simulink model "assemblage_19"  (R2016a)
settings: Solver=ode15s  StartTime=0.0  StopTime=1e6  RelTol=1e-3
undefined symbols (not defined in the file or in its folder): W
libraries: simCryogenics_lib x424, nesl_utility x343, fl_lib x9
(part 2 of 3)

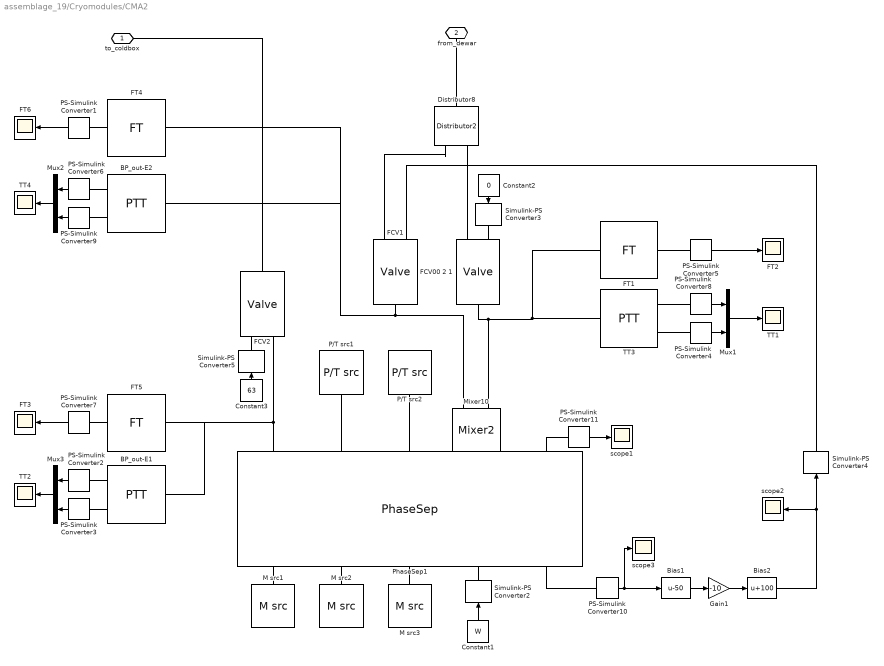
== system assemblage_19/Cryomodules/CMA2 ==
  BP_out-E1 : simCryogenics_lib/Sensors/PTT
  BP_out-E2 : simCryogenics_lib/Sensors/PTT
  Bias1 : Bias  Bias=-50
  Bias2 : Bias  Bias=100
  Constant1 : Constant  Value=W
  Constant2 : Constant  Value=0
  Constant3 : Constant  Value=63
  Distributor8 : simCryogenics_lib/Elements/Distributor2
  FCV00 2 1 : simCryogenics_lib/Elements/Valve  CVmax=0.2  ControlInputMin=0  ControlInputMax=100  Xt=0.86  Rv=100  lin_v=0  lim_v=0  K=2.4e-5 m^1.50000*kg^0.50000/s/bar^0.50000  Cmd_specify=off  Cmd_priority=High  Cmd=0  gamma_specify=off  gamma_priority=High  gamma=0  rho_specify=off  rho_priority=High  rho=0 kg/m^3  Xc_specify=off  Xc_priority=High  Xc=0  X_specify=off  X_priority=High  X=0  Y_specify=off  Y_priority=High  Y=0  CV_specify=off  CV_priority=High  CV=0
  FCV1 : simCryogenics_lib/Elements/Valve  CVmax=1.25  ControlInputMin=0  ControlInputMax=100  Xt=0.86  Rv=150  lin_v=0  lim_v=0  K=2.4e-5 m^1.50000*kg^0.50000/s/bar^0.50000  Cmd_specify=off  Cmd_priority=High  Cmd=0  gamma_specify=off  gamma_priority=High  gamma=0  rho_specify=off  rho_priority=High  rho=0 kg/m^3  Xc_specify=off  Xc_priority=High  Xc=0  X_specify=off  X_priority=High  X=0  Y_specify=off  Y_priority=High  Y=0  CV_specify=off  CV_priority=High  CV=0
  FCV2 : simCryogenics_lib/Elements/Valve  CVmax=1.5  ControlInputMin=0  ControlInputMax=100  Xt=0.86  Rv=100  lin_v=0  lim_v=0  K=2.4e-5 m^1.50000*kg^0.50000/s/bar^0.50000  Cmd_specify=off  Cmd_priority=High  Cmd=0  gamma_specify=off  gamma_priority=High  gamma=0  rho_specify=off  rho_priority=High  rho=0 kg/m^3  Xc_specify=off  Xc_priority=High  Xc=0  X_specify=off  X_priority=High  X=0  Y_specify=off  Y_priority=High  Y=0  CV_specify=off  CV_priority=High  CV=0
  FT1 : simCryogenics_lib/Sensors/FT
  FT2 : Scope
  FT3 : Scope
  FT4 : simCryogenics_lib/Sensors/FT
  FT5 : simCryogenics_lib/Sensors/FT
  FT6 : Scope
  Gain1 : Gain  Gain=-10
  M src1 : simCryogenics_lib/Sources_Sinks/M src  M=0 kg/s
  M src2 : simCryogenics_lib/Sources_Sinks/M src  M=0 kg/s
  M src3 : simCryogenics_lib/Sources_Sinks/M src  M=0 kg/s
  Mixer10 : simCryogenics_lib/Elements/Mixer2
  Mux1 : Mux  Inputs=2
  Mux2 : Mux  Inputs=2
  Mux3 : Mux  Inputs=2
  P/T src1 : simCryogenics_lib/Sources_Sinks/P//T src  P=1.2 bar  T=4.4 K
  P/T src2 : simCryogenics_lib/Sources_Sinks/P//T src  P=1.2 bar  T=4.4 K
  PS-Simulink Converter{1..11} (11 alike) : nesl_utility/PS-Simulink Converter  PhysicalDomain=network_engine_domain  SubClassName=ps_output  LeftPortType=input  RightPortType=output  PseudoPeriodic=off  Frequencies=[]  Unit=1  AffineConversion=off
  PhaseSep1 : simCryogenics_lib/Elements/PhaseSep  Ideal1=1  DeltaT1=0.05 K  N1=10  h1=400 W/K  Ideal2=1  DeltaT2=0.05 K  N2=10  h2=400 W/K  hmax=0.870 m  S=0.0402 m^2  P0=1.25 bar  h0=50  T0=4.5 K
  Simulink-PS Converter{2..5} (4 alike) : nesl_utility/Simulink-PS Converter  PhysicalDomain=network_engine_domain  SubClassName=ps_input  LeftPortType=input  RightPortType=output  PseudoPeriodic=off  Frequencies=[]  NoiseDistribution=none  NoiseParameters=[]  Unit=1  AffineConversion=off  InputFiltering=off  SimscapeFilterOrder=1  InputFilterTimeConstant=0.001  UdotUserProvided=1
  TT1 : Scope
  TT2 : Scope
  TT3 : simCryogenics_lib/Sensors/PTT
  TT4 : Scope
  scope1 : Scope
  scope2 : Scope
  scope3 : Scope
  to_coldbox : PMIOPort  Port=1  Side=Left
  from_dewar : PMIOPort  Port=2  Side=Right
  wires:
  PS-Simulink Converter5/1 -> FT2/1
  PS-Simulink Converter6/1 -> Mux2/1
  Mux3/1 -> TT2/1
  PS-Simulink Converter10/1 -> scope3/1, Bias1/1
  Constant3/1 -> Simulink-PS Converter5/1
  PS-Simulink Converter3/1 -> Mux3/2
  Constant2/1 -> Simulink-PS Converter3/1
  PS-Simulink Converter9/1 -> Mux2/2
  PS-Simulink Converter7/1 -> FT3/1
  PS-Simulink Converter1/1 -> FT6/1
  Gain1/1 -> Bias2/1
  PS-Simulink Converter11/1 -> scope1/1
  Mux2/1 -> TT4/1
  PS-Simulink Converter2/1 -> Mux3/1
  Mux1/1 -> TT1/1
  PS-Simulink Converter4/1 -> Mux1/2
  Bias2/1 -> scope2/1, Simulink-PS Converter4/1
  Constant1/1 -> Simulink-PS Converter2/1
  PS-Simulink Converter8/1 -> Mux1/1
  Bias1/1 -> Gain1/1
  connections:
  Simulink-PS Converter3/RConn1 -- FCV00 2 1/LConn1
  BP_out-E2/RConn2 -- PS-Simulink Converter6/LConn1
  PhaseSep1/RConn2 -- M src2/RConn1
  FCV1/RConn1 -- Mixer10/LConn2 -- FT4/LConn1 -- BP_out-E2/LConn1
  FT1/LConn1 -- TT3/LConn1 -- FCV00 2 1/RConn1 -- Mixer10/LConn1
  P/T src2/RConn1 -- PhaseSep1/LConn3
  TT3/RConn2 -- PS-Simulink Converter4/LConn1
  PS-Simulink Converter1/LConn1 -- FT4/RConn1
  FCV2/LConn1 -- Simulink-PS Converter5/RConn1
  Simulink-PS Converter2/RConn1 -- PhaseSep1/RConn4
  M src3/RConn1 -- PhaseSep1/RConn3
  FCV2/RConn1 -- to_coldbox/RConn1
  PhaseSep1/LConn2 -- P/T src1/RConn1
  FCV00 2 1/LConn2 -- Distributor8/RConn1
  BP_out-E1/RConn2 -- PS-Simulink Converter2/LConn1
  PhaseSep1/LConn4 -- Mixer10/RConn1
  PS-Simulink Converter10/LConn1 -- PhaseSep1/RConn5
  TT3/RConn1 -- PS-Simulink Converter8/LConn1
  FCV2/LConn2 -- PhaseSep1/LConn1 -- BP_out-E1/LConn1 -- FT5/LConn1
  from_dewar/RConn1 -- Distributor8/LConn1
  PS-Simulink Converter11/LConn1 -- PhaseSep1/LConn5
  M src1/RConn1 -- PhaseSep1/RConn1
  BP_out-E2/RConn1 -- PS-Simulink Converter9/LConn1
  PS-Simulink Converter5/LConn1 -- FT1/RConn1
  BP_out-E1/RConn1 -- PS-Simulink Converter3/LConn1
  Simulink-PS Converter4/RConn1 -- FCV1/LConn1
  PS-Simulink Converter7/LConn1 -- FT5/RConn1
  Distributor8/RConn2 -- FCV1/LConn2

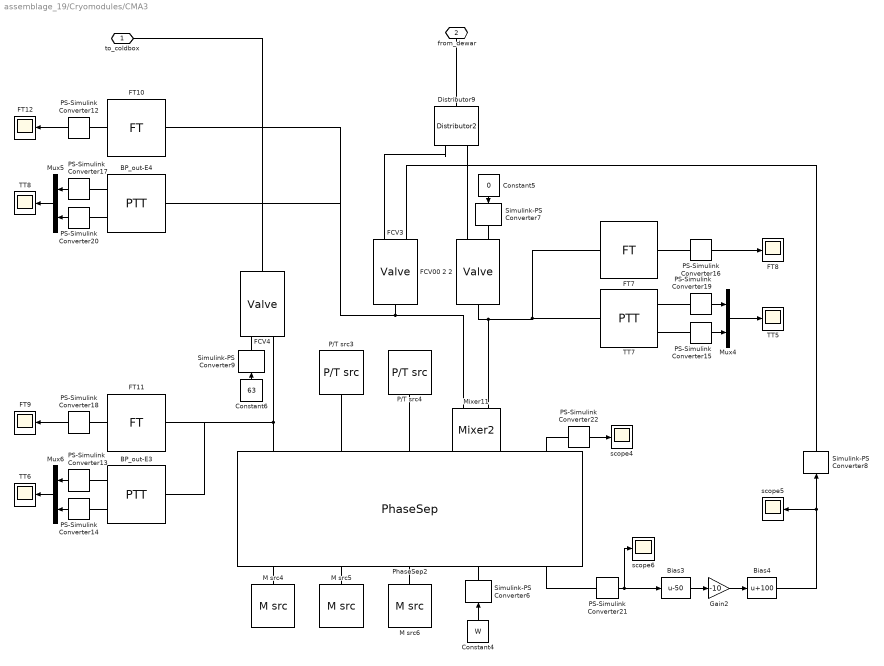
== system assemblage_19/Cryomodules/CMA3 ==
  BP_out-E3 : simCryogenics_lib/Sensors/PTT
  BP_out-E4 : simCryogenics_lib/Sensors/PTT
  Bias3 : Bias  Bias=-50
  Bias4 : Bias  Bias=100
  Constant4 : Constant  Value=W
  Constant5 : Constant  Value=0
  Constant6 : Constant  Value=63
  Distributor9 : simCryogenics_lib/Elements/Distributor2
  FCV00 2 2 : simCryogenics_lib/Elements/Valve  CVmax=0.2  ControlInputMin=0  ControlInputMax=100  Xt=0.86  Rv=100  lin_v=0  lim_v=0  K=2.4e-5 m^1.50000*kg^0.50000/s/bar^0.50000  Cmd_specify=off  Cmd_priority=High  Cmd=0  gamma_specify=off  gamma_priority=High  gamma=0  rho_specify=off  rho_priority=High  rho=0 kg/m^3  Xc_specify=off  Xc_priority=High  Xc=0  X_specify=off  X_priority=High  X=0  Y_specify=off  Y_priority=High  Y=0  CV_specify=off  CV_priority=High  CV=0
  FCV3 : simCryogenics_lib/Elements/Valve  CVmax=1.25  ControlInputMin=0  ControlInputMax=100  Xt=0.86  Rv=150  lin_v=0  lim_v=0  K=2.4e-5 m^1.50000*kg^0.50000/s/bar^0.50000  Cmd_specify=off  Cmd_priority=High  Cmd=0  gamma_specify=off  gamma_priority=High  gamma=0  rho_specify=off  rho_priority=High  rho=0 kg/m^3  Xc_specify=off  Xc_priority=High  Xc=0  X_specify=off  X_priority=High  X=0  Y_specify=off  Y_priority=High  Y=0  CV_specify=off  CV_priority=High  CV=0
  FCV4 : simCryogenics_lib/Elements/Valve  CVmax=1.5  ControlInputMin=0  ControlInputMax=100  Xt=0.86  Rv=100  lin_v=0  lim_v=0  K=2.4e-5 m^1.50000*kg^0.50000/s/bar^0.50000  Cmd_specify=off  Cmd_priority=High  Cmd=0  gamma_specify=off  gamma_priority=High  gamma=0  rho_specify=off  rho_priority=High  rho=0 kg/m^3  Xc_specify=off  Xc_priority=High  Xc=0  X_specify=off  X_priority=High  X=0  Y_specify=off  Y_priority=High  Y=0  CV_specify=off  CV_priority=High  CV=0
  FT10 : simCryogenics_lib/Sensors/FT
  FT11 : simCryogenics_lib/Sensors/FT
  FT12 : Scope
  FT7 : simCryogenics_lib/Sensors/FT
  FT8 : Scope
  FT9 : Scope
  Gain2 : Gain  Gain=-10
  M src4 : simCryogenics_lib/Sources_Sinks/M src  M=0 kg/s
  M src5 : simCryogenics_lib/Sources_Sinks/M src  M=0 kg/s
  M src6 : simCryogenics_lib/Sources_Sinks/M src  M=0 kg/s
  Mixer11 : simCryogenics_lib/Elements/Mixer2
  Mux4 : Mux  Inputs=2
  Mux5 : Mux  Inputs=2
  Mux6 : Mux  Inputs=2
  P/T src3 : simCryogenics_lib/Sources_Sinks/P//T src  P=1.2 bar  T=4.4 K
  P/T src4 : simCryogenics_lib/Sources_Sinks/P//T src  P=1.2 bar  T=4.4 K
  PS-Simulink Converter{12..22} (11 alike) : nesl_utility/PS-Simulink Converter  PhysicalDomain=network_engine_domain  SubClassName=ps_output  LeftPortType=input  RightPortType=output  PseudoPeriodic=off  Frequencies=[]  Unit=1  AffineConversion=off
  PhaseSep2 : simCryogenics_lib/Elements/PhaseSep  Ideal1=1  DeltaT1=0.05 K  N1=10  h1=400 W/K  Ideal2=1  DeltaT2=0.05 K  N2=10  h2=400 W/K  hmax=0.870 m  S=0.0402 m^2  P0=1.25 bar  h0=50  T0=4.5 K
  Simulink-PS Converter{6..9} (4 alike) : nesl_utility/Simulink-PS Converter  PhysicalDomain=network_engine_domain  SubClassName=ps_input  LeftPortType=input  RightPortType=output  PseudoPeriodic=off  Frequencies=[]  NoiseDistribution=none  NoiseParameters=[]  Unit=1  AffineConversion=off  InputFiltering=off  SimscapeFilterOrder=1  InputFilterTimeConstant=0.001  UdotUserProvided=1
  TT5 : Scope
  TT6 : Scope
  TT7 : simCryogenics_lib/Sensors/PTT
  TT8 : Scope
  scope4 : Scope
  scope5 : Scope
  scope6 : Scope
  to_coldbox : PMIOPort  Port=1  Side=Left
  from_dewar : PMIOPort  Port=2  Side=Right
  wires:
  PS-Simulink Converter16/1 -> FT8/1
  Mux6/1 -> TT6/1
  PS-Simulink Converter18/1 -> FT9/1
  PS-Simulink Converter20/1 -> Mux5/2
  PS-Simulink Converter17/1 -> Mux5/1
  Bias4/1 -> scope5/1, Simulink-PS Converter8/1
  Gain2/1 -> Bias4/1
  PS-Simulink Converter14/1 -> Mux6/2
  Constant4/1 -> Simulink-PS Converter6/1
  Constant5/1 -> Simulink-PS Converter7/1
  PS-Simulink Converter19/1 -> Mux4/1
  PS-Simulink Converter13/1 -> Mux6/1
  PS-Simulink Converter12/1 -> FT12/1
  Constant6/1 -> Simulink-PS Converter9/1
  PS-Simulink Converter22/1 -> scope4/1
  PS-Simulink Converter21/1 -> scope6/1, Bias3/1
  Mux4/1 -> TT5/1
  PS-Simulink Converter15/1 -> Mux4/2
  Mux5/1 -> TT8/1
  Bias3/1 -> Gain2/1
  connections:
  BP_out-E4/RConn2 -- PS-Simulink Converter17/LConn1
  FCV4/LConn1 -- Simulink-PS Converter9/RConn1
  BP_out-E3/RConn2 -- PS-Simulink Converter13/LConn1
  FT7/LConn1 -- TT7/LConn1 -- FCV00 2 2/RConn1 -- Mixer11/LConn1
  PS-Simulink Converter18/LConn1 -- FT11/RConn1
  from_dewar/RConn1 -- Distributor9/LConn1
  FCV00 2 2/LConn2 -- Distributor9/RConn1
  PhaseSep2/LConn2 -- P/T src3/RConn1
  FCV3/RConn1 -- Mixer11/LConn2 -- FT10/LConn1 -- BP_out-E4/LConn1
  Simulink-PS Converter6/RConn1 -- PhaseSep2/RConn4
  Simulink-PS Converter7/RConn1 -- FCV00 2 2/LConn1
  FCV4/RConn1 -- to_coldbox/RConn1
  PhaseSep2/RConn2 -- M src5/RConn1
  M src4/RConn1 -- PhaseSep2/RConn1
  FCV4/LConn2 -- PhaseSep2/LConn1 -- BP_out-E3/LConn1 -- FT11/LConn1
  Simulink-PS Converter8/RConn1 -- FCV3/LConn1
  PS-Simulink Converter22/LConn1 -- PhaseSep2/LConn5
  Distributor9/RConn2 -- FCV3/LConn2
  P/T src4/RConn1 -- PhaseSep2/LConn3
  TT7/RConn2 -- PS-Simulink Converter15/LConn1
  TT7/RConn1 -- PS-Simulink Converter19/LConn1
  PS-Simulink Converter16/LConn1 -- FT7/RConn1
  BP_out-E3/RConn1 -- PS-Simulink Converter14/LConn1
  M src6/RConn1 -- PhaseSep2/RConn3
  PS-Simulink Converter12/LConn1 -- FT10/RConn1
  PS-Simulink Converter21/LConn1 -- PhaseSep2/RConn5
  PhaseSep2/LConn4 -- Mixer11/RConn1
  BP_out-E4/RConn1 -- PS-Simulink Converter20/LConn1

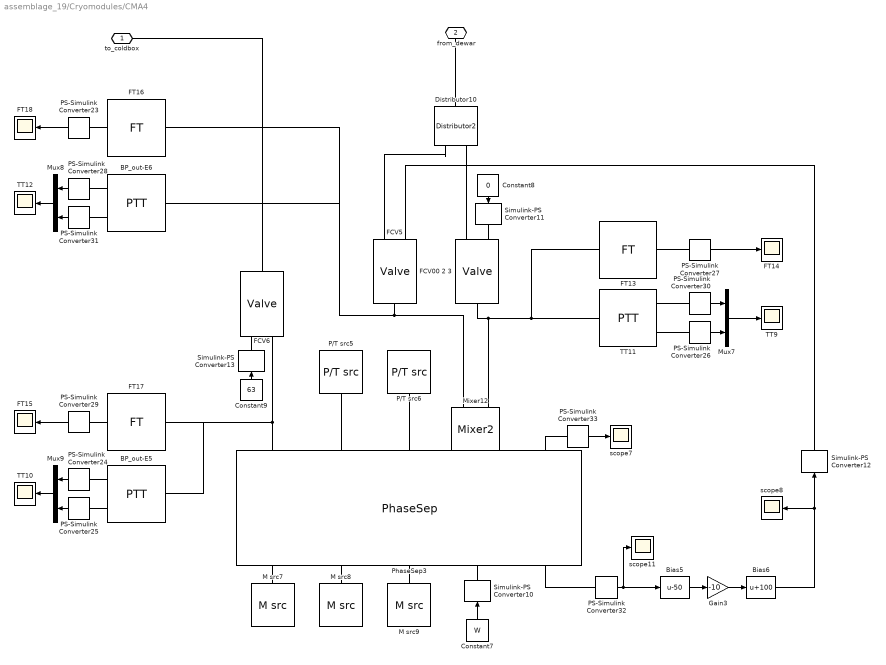
== system assemblage_19/Cryomodules/CMA4 ==
  BP_out-E5 : simCryogenics_lib/Sensors/PTT
  BP_out-E6 : simCryogenics_lib/Sensors/PTT
  Bias5 : Bias  Bias=-50
  Bias6 : Bias  Bias=100
  Constant7 : Constant  Value=W
  Constant8 : Constant  Value=0
  Constant9 : Constant  Value=63
  Distributor10 : simCryogenics_lib/Elements/Distributor2
  FCV00 2 3 : simCryogenics_lib/Elements/Valve  CVmax=0.2  ControlInputMin=0  ControlInputMax=100  Xt=0.86  Rv=100  lin_v=0  lim_v=0  K=2.4e-5 m^1.50000*kg^0.50000/s/bar^0.50000  Cmd_specify=off  Cmd_priority=High  Cmd=0  gamma_specify=off  gamma_priority=High  gamma=0  rho_specify=off  rho_priority=High  rho=0 kg/m^3  Xc_specify=off  Xc_priority=High  Xc=0  X_specify=off  X_priority=High  X=0  Y_specify=off  Y_priority=High  Y=0  CV_specify=off  CV_priority=High  CV=0
  FCV5 : simCryogenics_lib/Elements/Valve  CVmax=1.25  ControlInputMin=0  ControlInputMax=100  Xt=0.86  Rv=150  lin_v=0  lim_v=0  K=2.4e-5 m^1.50000*kg^0.50000/s/bar^0.50000  Cmd_specify=off  Cmd_priority=High  Cmd=0  gamma_specify=off  gamma_priority=High  gamma=0  rho_specify=off  rho_priority=High  rho=0 kg/m^3  Xc_specify=off  Xc_priority=High  Xc=0  X_specify=off  X_priority=High  X=0  Y_specify=off  Y_priority=High  Y=0  CV_specify=off  CV_priority=High  CV=0
  FCV6 : simCryogenics_lib/Elements/Valve  CVmax=1.5  ControlInputMin=0  ControlInputMax=100  Xt=0.86  Rv=100  lin_v=0  lim_v=0  K=2.4e-5 m^1.50000*kg^0.50000/s/bar^0.50000  Cmd_specify=off  Cmd_priority=High  Cmd=0  gamma_specify=off  gamma_priority=High  gamma=0  rho_specify=off  rho_priority=High  rho=0 kg/m^3  Xc_specify=off  Xc_priority=High  Xc=0  X_specify=off  X_priority=High  X=0  Y_specify=off  Y_priority=High  Y=0  CV_specify=off  CV_priority=High  CV=0
  FT13 : simCryogenics_lib/Sensors/FT
  FT14 : Scope
  FT15 : Scope
  FT16 : simCryogenics_lib/Sensors/FT
  FT17 : simCryogenics_lib/Sensors/FT
  FT18 : Scope
  Gain3 : Gain  Gain=-10
  M src7 : simCryogenics_lib/Sources_Sinks/M src  M=0 kg/s
  M src8 : simCryogenics_lib/Sources_Sinks/M src  M=0 kg/s
  M src9 : simCryogenics_lib/Sources_Sinks/M src  M=0 kg/s
  Mixer12 : simCryogenics_lib/Elements/Mixer2
  Mux7 : Mux  Inputs=2
  Mux8 : Mux  Inputs=2
  Mux9 : Mux  Inputs=2
  P/T src5 : simCryogenics_lib/Sources_Sinks/P//T src  P=1.2 bar  T=4.4 K
  P/T src6 : simCryogenics_lib/Sources_Sinks/P//T src  P=1.2 bar  T=4.4 K
  PS-Simulink Converter{23..33} (11 alike) : nesl_utility/PS-Simulink Converter  PhysicalDomain=network_engine_domain  SubClassName=ps_output  LeftPortType=input  RightPortType=output  PseudoPeriodic=off  Frequencies=[]  Unit=1  AffineConversion=off
  PhaseSep3 : simCryogenics_lib/Elements/PhaseSep  Ideal1=1  DeltaT1=0.05 K  N1=10  h1=400 W/K  Ideal2=1  DeltaT2=0.05 K  N2=10  h2=400 W/K  hmax=0.870 m  S=0.0402 m^2  P0=1.25 bar  h0=50  T0=4.5 K
  Simulink-PS Converter{10..13} (4 alike) : nesl_utility/Simulink-PS Converter  PhysicalDomain=network_engine_domain  SubClassName=ps_input  LeftPortType=input  RightPortType=output  PseudoPeriodic=off  Frequencies=[]  NoiseDistribution=none  NoiseParameters=[]  Unit=1  AffineConversion=off  InputFiltering=off  SimscapeFilterOrder=1  InputFilterTimeConstant=0.001  UdotUserProvided=1
  TT10 : Scope
  TT11 : simCryogenics_lib/Sensors/PTT
  TT12 : Scope
  TT9 : Scope
  scope11 : Scope
  scope7 : Scope
  scope8 : Scope
  to_coldbox : PMIOPort  Port=1  Side=Left
  from_dewar : PMIOPort  Port=2  Side=Right
  wires:
  PS-Simulink Converter25/1 -> Mux9/2
  PS-Simulink Converter30/1 -> Mux7/1
  PS-Simulink Converter28/1 -> Mux8/1
  PS-Simulink Converter32/1 -> scope11/1, Bias5/1
  PS-Simulink Converter27/1 -> FT14/1
  PS-Simulink Converter33/1 -> scope7/1
  Mux8/1 -> TT12/1
  PS-Simulink Converter26/1 -> Mux7/2
  Gain3/1 -> Bias6/1
  PS-Simulink Converter23/1 -> FT18/1
  Constant9/1 -> Simulink-PS Converter13/1
  Bias5/1 -> Gain3/1
  PS-Simulink Converter29/1 -> FT15/1
  Mux7/1 -> TT9/1
  PS-Simulink Converter31/1 -> Mux8/2
  Mux9/1 -> TT10/1
  PS-Simulink Converter24/1 -> Mux9/1
  Constant8/1 -> Simulink-PS Converter11/1
  Constant7/1 -> Simulink-PS Converter10/1
  Bias6/1 -> scope8/1, Simulink-PS Converter12/1
  connections:
  Simulink-PS Converter11/RConn1 -- FCV00 2 3/LConn1
  FCV6/RConn1 -- to_coldbox/RConn1
  FCV6/LConn1 -- Simulink-PS Converter13/RConn1
  P/T src6/RConn1 -- PhaseSep3/LConn3
  PhaseSep3/LConn4 -- Mixer12/RConn1
  Simulink-PS Converter10/RConn1 -- PhaseSep3/RConn4
  Distributor10/RConn2 -- FCV5/LConn2
  FCV6/LConn2 -- PhaseSep3/LConn1 -- BP_out-E5/LConn1 -- FT17/LConn1
  BP_out-E6/RConn1 -- PS-Simulink Converter31/LConn1
  FCV5/RConn1 -- Mixer12/LConn2 -- FT16/LConn1 -- BP_out-E6/LConn1
  M src7/RConn1 -- PhaseSep3/RConn1
  BP_out-E5/RConn1 -- PS-Simulink Converter25/LConn1
  PS-Simulink Converter32/LConn1 -- PhaseSep3/RConn5
  TT11/RConn1 -- PS-Simulink Converter30/LConn1
  PS-Simulink Converter23/LConn1 -- FT16/RConn1
  BP_out-E5/RConn2 -- PS-Simulink Converter24/LConn1
  TT11/RConn2 -- PS-Simulink Converter26/LConn1
  PS-Simulink Converter27/LConn1 -- FT13/RConn1
  FCV00 2 3/LConn2 -- Distributor10/RConn1
  from_dewar/RConn1 -- Distributor10/LConn1
  FT13/LConn1 -- TT11/LConn1 -- FCV00 2 3/RConn1 -- Mixer12/LConn1
  PhaseSep3/RConn2 -- M src8/RConn1
  PhaseSep3/LConn2 -- P/T src5/RConn1
  Simulink-PS Converter12/RConn1 -- FCV5/LConn1
  BP_out-E6/RConn2 -- PS-Simulink Converter28/LConn1
  M src9/RConn1 -- PhaseSep3/RConn3
  PS-Simulink Converter29/LConn1 -- FT17/RConn1
  PS-Simulink Converter33/LConn1 -- PhaseSep3/LConn5

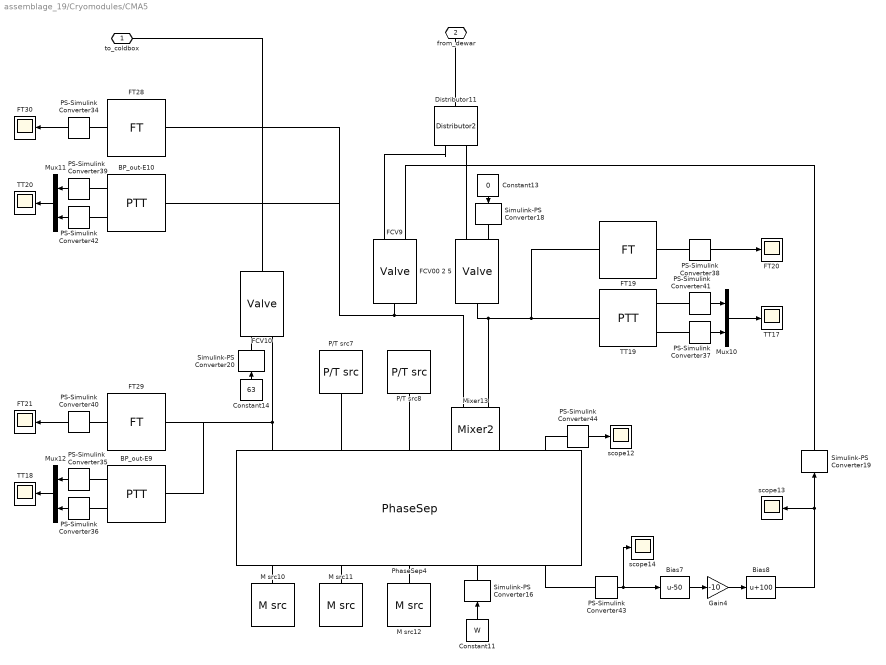
== system assemblage_19/Cryomodules/CMA5 ==
  BP_out-E10 : simCryogenics_lib/Sensors/PTT
  BP_out-E9 : simCryogenics_lib/Sensors/PTT
  Bias7 : Bias  Bias=-50
  Bias8 : Bias  Bias=100
  Constant11 : Constant  Value=W
  Constant13 : Constant  Value=0
  Constant14 : Constant  Value=63
  Distributor11 : simCryogenics_lib/Elements/Distributor2
  FCV00 2 5 : simCryogenics_lib/Elements/Valve  CVmax=0.2  ControlInputMin=0  ControlInputMax=100  Xt=0.86  Rv=100  lin_v=0  lim_v=0  K=2.4e-5 m^1.50000*kg^0.50000/s/bar^0.50000  Cmd_specify=off  Cmd_priority=High  Cmd=0  gamma_specify=off  gamma_priority=High  gamma=0  rho_specify=off  rho_priority=High  rho=0 kg/m^3  Xc_specify=off  Xc_priority=High  Xc=0  X_specify=off  X_priority=High  X=0  Y_specify=off  Y_priority=High  Y=0  CV_specify=off  CV_priority=High  CV=0
  FCV10 : simCryogenics_lib/Elements/Valve  CVmax=1.5  ControlInputMin=0  ControlInputMax=100  Xt=0.86  Rv=100  lin_v=0  lim_v=0  K=2.4e-5 m^1.50000*kg^0.50000/s/bar^0.50000  Cmd_specify=off  Cmd_priority=High  Cmd=0  gamma_specify=off  gamma_priority=High  gamma=0  rho_specify=off  rho_priority=High  rho=0 kg/m^3  Xc_specify=off  Xc_priority=High  Xc=0  X_specify=off  X_priority=High  X=0  Y_specify=off  Y_priority=High  Y=0  CV_specify=off  CV_priority=High  CV=0
  FCV9 : simCryogenics_lib/Elements/Valve  CVmax=1.25  ControlInputMin=0  ControlInputMax=100  Xt=0.86  Rv=150  lin_v=0  lim_v=0  K=2.4e-5 m^1.50000*kg^0.50000/s/bar^0.50000  Cmd_specify=off  Cmd_priority=High  Cmd=0  gamma_specify=off  gamma_priority=High  gamma=0  rho_specify=off  rho_priority=High  rho=0 kg/m^3  Xc_specify=off  Xc_priority=High  Xc=0  X_specify=off  X_priority=High  X=0  Y_specify=off  Y_priority=High  Y=0  CV_specify=off  CV_priority=High  CV=0
  FT19 : simCryogenics_lib/Sensors/FT
  FT20 : Scope
  FT21 : Scope
  FT28 : simCryogenics_lib/Sensors/FT
  FT29 : simCryogenics_lib/Sensors/FT
  FT30 : Scope
  Gain4 : Gain  Gain=-10
  M src10 : simCryogenics_lib/Sources_Sinks/M src  M=0 kg/s
  M src11 : simCryogenics_lib/Sources_Sinks/M src  M=0 kg/s
  M src12 : simCryogenics_lib/Sources_Sinks/M src  M=0 kg/s
  Mixer13 : simCryogenics_lib/Elements/Mixer2
  Mux10 : Mux  Inputs=2
  Mux11 : Mux  Inputs=2
  Mux12 : Mux  Inputs=2
  P/T src7 : simCryogenics_lib/Sources_Sinks/P//T src  P=1.2 bar  T=4.4 K
  P/T src8 : simCryogenics_lib/Sources_Sinks/P//T src  P=1.2 bar  T=4.4 K
  PS-Simulink Converter{34..44} (11 alike) : nesl_utility/PS-Simulink Converter  PhysicalDomain=network_engine_domain  SubClassName=ps_output  LeftPortType=input  RightPortType=output  PseudoPeriodic=off  Frequencies=[]  Unit=1  AffineConversion=off
  PhaseSep4 : simCryogenics_lib/Elements/PhaseSep  Ideal1=1  DeltaT1=0.05 K  N1=10  h1=400 W/K  Ideal2=1  DeltaT2=0.05 K  N2=10  h2=400 W/K  hmax=0.870 m  S=0.0402 m^2  P0=1.25 bar  h0=50  T0=4.5 K
  Simulink-PS Converter{16,18..20} (4 alike) : nesl_utility/Simulink-PS Converter  PhysicalDomain=network_engine_domain  SubClassName=ps_input  LeftPortType=input  RightPortType=output  PseudoPeriodic=off  Frequencies=[]  NoiseDistribution=none  NoiseParameters=[]  Unit=1  AffineConversion=off  InputFiltering=off  SimscapeFilterOrder=1  InputFilterTimeConstant=0.001  UdotUserProvided=1
  TT17 : Scope
  TT18 : Scope
  TT19 : simCryogenics_lib/Sensors/PTT
  TT20 : Scope
  scope12 : Scope
  scope13 : Scope
  scope14 : Scope
  to_coldbox : PMIOPort  Port=1  Side=Left
  from_dewar : PMIOPort  Port=2  Side=Right
  wires:
  PS-Simulink Converter34/1 -> FT30/1
  Gain4/1 -> Bias8/1
  PS-Simulink Converter41/1 -> Mux10/1
  Constant13/1 -> Simulink-PS Converter18/1
  PS-Simulink Converter42/1 -> Mux11/2
  Bias8/1 -> scope13/1, Simulink-PS Converter19/1
  PS-Simulink Converter44/1 -> scope12/1
  PS-Simulink Converter40/1 -> FT21/1
  PS-Simulink Converter38/1 -> FT20/1
  Mux12/1 -> TT18/1
  Constant14/1 -> Simulink-PS Converter20/1
  Constant11/1 -> Simulink-PS Converter16/1
  PS-Simulink Converter36/1 -> Mux12/2
  PS-Simulink Converter43/1 -> scope14/1, Bias7/1
  PS-Simulink Converter39/1 -> Mux11/1
  Bias7/1 -> Gain4/1
  Mux11/1 -> TT20/1
  PS-Simulink Converter35/1 -> Mux12/1
  Mux10/1 -> TT17/1
  PS-Simulink Converter37/1 -> Mux10/2
  connections:
  FCV00 2 5/LConn2 -- Distributor11/RConn1
  BP_out-E9/RConn2 -- PS-Simulink Converter35/LConn1
  M src12/RConn1 -- PhaseSep4/RConn3
  FCV10/RConn1 -- to_coldbox/RConn1
  Simulink-PS Converter18/RConn1 -- FCV00 2 5/LConn1
  BP_out-E10/RConn2 -- PS-Simulink Converter39/LConn1
  PhaseSep4/LConn4 -- Mixer13/RConn1
  from_dewar/RConn1 -- Distributor11/LConn1
  TT19/RConn1 -- PS-Simulink Converter41/LConn1
  PhaseSep4/RConn2 -- M src11/RConn1
  BP_out-E9/RConn1 -- PS-Simulink Converter36/LConn1
  PS-Simulink Converter44/LConn1 -- PhaseSep4/LConn5
  Distributor11/RConn2 -- FCV9/LConn2
  BP_out-E10/RConn1 -- PS-Simulink Converter42/LConn1
  FCV10/LConn1 -- Simulink-PS Converter20/RConn1
  PS-Simulink Converter43/LConn1 -- PhaseSep4/RConn5
  PS-Simulink Converter34/LConn1 -- FT28/RConn1
  Simulink-PS Converter16/RConn1 -- PhaseSep4/RConn4
  FCV9/RConn1 -- Mixer13/LConn2 -- FT28/LConn1 -- BP_out-E10/LConn1
  TT19/RConn2 -- PS-Simulink Converter37/LConn1
  P/T src8/RConn1 -- PhaseSep4/LConn3
  FCV10/LConn2 -- PhaseSep4/LConn1 -- BP_out-E9/LConn1 -- FT29/LConn1
  PS-Simulink Converter40/LConn1 -- FT29/RConn1
  Simulink-PS Converter19/RConn1 -- FCV9/LConn1
  M src10/RConn1 -- PhaseSep4/RConn1
  PS-Simulink Converter38/LConn1 -- FT19/RConn1
  PhaseSep4/LConn2 -- P/T src7/RConn1
  FT19/LConn1 -- TT19/LConn1 -- FCV00 2 5/RConn1 -- Mixer13/LConn1

== system assemblage_19/Cryomodules/CMA6 ==
  BP_out-E11 : simCryogenics_lib/Sensors/PTT
  BP_out-E12 : simCryogenics_lib/Sensors/PTT
  Bias11 : Bias  Bias=-50
  Bias12 : Bias  Bias=100
  Constant15 : Constant  Value=W
  Constant16 : Constant  Value=0
  Constant17 : Constant  Value=63
  Distributor12 : simCryogenics_lib/Elements/Distributor2
  FCV00 2 6 : simCryogenics_lib/Elements/Valve  CVmax=0.2  ControlInputMin=0  ControlInputMax=100  Xt=0.86  Rv=100  lin_v=0  lim_v=0  K=2.4e-5 m^1.50000*kg^0.50000/s/bar^0.50000  Cmd_specify=off  Cmd_priority=High  Cmd=0  gamma_specify=off  gamma_priority=High  gamma=0  rho_specify=off  rho_priority=High  rho=0 kg/m^3  Xc_specify=off  Xc_priority=High  Xc=0  X_specify=off  X_priority=High  X=0  Y_specify=off  Y_priority=High  Y=0  CV_specify=off  CV_priority=High  CV=0
  FCV11 : simCryogenics_lib/Elements/Valve  CVmax=1.25  ControlInputMin=0  ControlInputMax=100  Xt=0.86  Rv=150  lin_v=0  lim_v=0  K=2.4e-5 m^1.50000*kg^0.50000/s/bar^0.50000  Cmd_specify=off  Cmd_priority=High  Cmd=0  gamma_specify=off  gamma_priority=High  gamma=0  rho_specify=off  rho_priority=High  rho=0 kg/m^3  Xc_specify=off  Xc_priority=High  Xc=0  X_specify=off  X_priority=High  X=0  Y_specify=off  Y_priority=High  Y=0  CV_specify=off  CV_priority=High  CV=0
  FCV12 : simCryogenics_lib/Elements/Valve  CVmax=1.5  ControlInputMin=0  ControlInputMax=100  Xt=0.86  Rv=100  lin_v=0  lim_v=0  K=2.4e-5 m^1.50000*kg^0.50000/s/bar^0.50000  Cmd_specify=off  Cmd_priority=High  Cmd=0  gamma_specify=off  gamma_priority=High  gamma=0  rho_specify=off  rho_priority=High  rho=0 kg/m^3  Xc_specify=off  Xc_priority=High  Xc=0  X_specify=off  X_priority=High  X=0  Y_specify=off  Y_priority=High  Y=0  CV_specify=off  CV_priority=High  CV=0
  FT31 : simCryogenics_lib/Sensors/FT
  FT32 : Scope
  FT33 : Scope
  FT34 : simCryogenics_lib/Sensors/FT
  FT35 : simCryogenics_lib/Sensors/FT
  FT36 : Scope
  Gain6 : Gain  Gain=-10
  M src16 : simCryogenics_lib/Sources_Sinks/M src  M=0 kg/s
  M src17 : simCryogenics_lib/Sources_Sinks/M src  M=0 kg/s
  M src18 : simCryogenics_lib/Sources_Sinks/M src  M=0 kg/s
  Mixer14 : simCryogenics_lib/Elements/Mixer2
  Mux13 : Mux  Inputs=2
  Mux14 : Mux  Inputs=2
  Mux15 : Mux  Inputs=2
  P/T src10 : simCryogenics_lib/Sources_Sinks/P//T src  P=1.2 bar  T=4.4 K
  P/T src9 : simCryogenics_lib/Sources_Sinks/P//T src  P=1.2 bar  T=4.4 K
  PS-Simulink Converter{45..55} (11 alike) : nesl_utility/PS-Simulink Converter  PhysicalDomain=network_engine_domain  SubClassName=ps_output  LeftPortType=input  RightPortType=output  PseudoPeriodic=off  Frequencies=[]  Unit=1  AffineConversion=off
  PhaseSep6 : simCryogenics_lib/Elements/PhaseSep  Ideal1=1  DeltaT1=0.05 K  N1=10  h1=400 W/K  Ideal2=1  DeltaT2=0.05 K  N2=10  h2=400 W/K  hmax=0.870 m  S=0.0402 m^2  P0=1.25 bar  h0=50  T0=4.5 K
  Simulink-PS Converter{21..24} (4 alike) : nesl_utility/Simulink-PS Converter  PhysicalDomain=network_engine_domain  SubClassName=ps_input  LeftPortType=input  RightPortType=output  PseudoPeriodic=off  Frequencies=[]  NoiseDistribution=none  NoiseParameters=[]  Unit=1  AffineConversion=off  InputFiltering=off  SimscapeFilterOrder=1  InputFilterTimeConstant=0.001  UdotUserProvided=1
  TT21 : Scope
  TT22 : Scope
  TT23 : simCryogenics_lib/Sensors/PTT
  TT24 : Scope
  scope16 : Scope
  scope17 : Scope
  scope18 : Scope
  to_coldbox : PMIOPort  Port=1  Side=Left
  from_dewar : PMIOPort  Port=2  Side=Right
  wires:
  Bias12/1 -> scope17/1, Simulink-PS Converter23/1
  Mux15/1 -> TT22/1
  Mux13/1 -> TT21/1
  Mux14/1 -> TT24/1
  PS-Simulink Converter52/1 -> Mux13/1
  PS-Simulink Converter45/1 -> FT36/1
  PS-Simulink Converter55/1 -> scope16/1
  PS-Simulink Converter49/1 -> FT32/1
  PS-Simulink Converter54/1 -> scope18/1, Bias11/1
  Constant16/1 -> Simulink-PS Converter22/1
  PS-Simulink Converter50/1 -> Mux14/1
  PS-Simulink Converter47/1 -> Mux15/2
  Constant17/1 -> Simulink-PS Converter24/1
  Bias11/1 -> Gain6/1
  PS-Simulink Converter53/1 -> Mux14/2
  PS-Simulink Converter48/1 -> Mux13/2
  PS-Simulink Converter46/1 -> Mux15/1
  Gain6/1 -> Bias12/1
  PS-Simulink Converter51/1 -> FT33/1
  Constant15/1 -> Simulink-PS Converter21/1
  connections:
  M src16/RConn1 -- PhaseSep6/RConn1
  FCV12/LConn1 -- Simulink-PS Converter24/RConn1
  BP_out-E12/RConn2 -- PS-Simulink Converter50/LConn1
  PhaseSep6/RConn2 -- M src17/RConn1
  FCV12/RConn1 -- to_coldbox/RConn1
  M src18/RConn1 -- PhaseSep6/RConn3
  PhaseSep6/LConn4 -- Mixer14/RConn1
  PhaseSep6/LConn2 -- P/T src9/RConn1
  from_dewar/RConn1 -- Distributor12/LConn1
  PS-Simulink Converter55/LConn1 -- PhaseSep6/LConn5
  PS-Simulink Converter51/LConn1 -- FT35/RConn1
  TT23/RConn1 -- PS-Simulink Converter52/LConn1
  Simulink-PS Converter21/RConn1 -- PhaseSep6/RConn4
  BP_out-E11/RConn2 -- PS-Simulink Converter46/LConn1
  PS-Simulink Converter54/LConn1 -- PhaseSep6/RConn5
  FCV00 2 6/LConn2 -- Distributor12/RConn1
  PS-Simulink Converter45/LConn1 -- FT34/RConn1
  FCV12/LConn2 -- PhaseSep6/LConn1 -- BP_out-E11/LConn1 -- FT35/LConn1
  TT23/RConn2 -- PS-Simulink Converter48/LConn1
  FCV11/RConn1 -- Mixer14/LConn2 -- FT34/LConn1 -- BP_out-E12/LConn1
  FT31/LConn1 -- TT23/LConn1 -- FCV00 2 6/RConn1 -- Mixer14/LConn1
  P/T src10/RConn1 -- PhaseSep6/LConn3
  Simulink-PS Converter22/RConn1 -- FCV00 2 6/LConn1
  BP_out-E12/RConn1 -- PS-Simulink Converter53/LConn1
  Simulink-PS Converter23/RConn1 -- FCV11/LConn1
  Distributor12/RConn2 -- FCV11/LConn2
  BP_out-E11/RConn1 -- PS-Simulink Converter47/LConn1
  PS-Simulink Converter49/LConn1 -- FT31/RConn1

== system assemblage_19/Cryomodules/CMA7 ==
  BP_out-E13 : simCryogenics_lib/Sensors/PTT
  BP_out-E14 : simCryogenics_lib/Sensors/PTT
  Bias13 : Bias  Bias=-50
  Bias14 : Bias  Bias=100
  Constant18 : Constant  Value=W
  Constant19 : Constant  Value=0
  Constant20 : Constant  Value=63
  Distributor13 : simCryogenics_lib/Elements/Distributor2
  FCV00 2 7 : simCryogenics_lib/Elements/Valve  CVmax=0.2  ControlInputMin=0  ControlInputMax=100  Xt=0.86  Rv=100  lin_v=0  lim_v=0  K=2.4e-5 m^1.50000*kg^0.50000/s/bar^0.50000  Cmd_specify=off  Cmd_priority=High  Cmd=0  gamma_specify=off  gamma_priority=High  gamma=0  rho_specify=off  rho_priority=High  rho=0 kg/m^3  Xc_specify=off  Xc_priority=High  Xc=0  X_specify=off  X_priority=High  X=0  Y_specify=off  Y_priority=High  Y=0  CV_specify=off  CV_priority=High  CV=0
  FCV13 : simCryogenics_lib/Elements/Valve  CVmax=1.25  ControlInputMin=0  ControlInputMax=100  Xt=0.86  Rv=150  lin_v=0  lim_v=0  K=2.4e-5 m^1.50000*kg^0.50000/s/bar^0.50000  Cmd_specify=off  Cmd_priority=High  Cmd=0  gamma_specify=off  gamma_priority=High  gamma=0  rho_specify=off  rho_priority=High  rho=0 kg/m^3  Xc_specify=off  Xc_priority=High  Xc=0  X_specify=off  X_priority=High  X=0  Y_specify=off  Y_priority=High  Y=0  CV_specify=off  CV_priority=High  CV=0
  FCV14 : simCryogenics_lib/Elements/Valve  CVmax=1.5  ControlInputMin=0  ControlInputMax=100  Xt=0.86  Rv=100  lin_v=0  lim_v=0  K=2.4e-5 m^1.50000*kg^0.50000/s/bar^0.50000  Cmd_specify=off  Cmd_priority=High  Cmd=0  gamma_specify=off  gamma_priority=High  gamma=0  rho_specify=off  rho_priority=High  rho=0 kg/m^3  Xc_specify=off  Xc_priority=High  Xc=0  X_specify=off  X_priority=High  X=0  Y_specify=off  Y_priority=High  Y=0  CV_specify=off  CV_priority=High  CV=0
  FT37 : simCryogenics_lib/Sensors/FT
  FT38 : Scope
  FT39 : Scope
  FT40 : simCryogenics_lib/Sensors/FT
  FT41 : simCryogenics_lib/Sensors/FT
  FT42 : Scope
  Gain7 : Gain  Gain=-10
  M src19 : simCryogenics_lib/Sources_Sinks/M src  M=0 kg/s
  M src20 : simCryogenics_lib/Sources_Sinks/M src  M=0 kg/s
  M src21 : simCryogenics_lib/Sources_Sinks/M src  M=0 kg/s
  Mixer15 : simCryogenics_lib/Elements/Mixer2
  Mux16 : Mux  Inputs=2
  Mux17 : Mux  Inputs=2
  Mux18 : Mux  Inputs=2
  P/T src11 : simCryogenics_lib/Sources_Sinks/P//T src  P=1.2 bar  T=4.4 K
  P/T src12 : simCryogenics_lib/Sources_Sinks/P//T src  P=1.2 bar  T=4.4 K
  PS-Simulink Converter{56..66} (11 alike) : nesl_utility/PS-Simulink Converter  PhysicalDomain=network_engine_domain  SubClassName=ps_output  LeftPortType=input  RightPortType=output  PseudoPeriodic=off  Frequencies=[]  Unit=1  AffineConversion=off
  PhaseSep7 : simCryogenics_lib/Elements/PhaseSep  Ideal1=1  DeltaT1=0.05 K  N1=10  h1=400 W/K  Ideal2=1  DeltaT2=0.05 K  N2=10  h2=400 W/K  hmax=0.870 m  S=0.0402 m^2  P0=1.25 bar  h0=50  T0=4.5 K
  Simulink-PS Converter{25..28} (4 alike) : nesl_utility/Simulink-PS Converter  PhysicalDomain=network_engine_domain  SubClassName=ps_input  LeftPortType=input  RightPortType=output  PseudoPeriodic=off  Frequencies=[]  NoiseDistribution=none  NoiseParameters=[]  Unit=1  AffineConversion=off  InputFiltering=off  SimscapeFilterOrder=1  InputFilterTimeConstant=0.001  UdotUserProvided=1
  TT25 : Scope
  TT26 : Scope
  TT27 : simCryogenics_lib/Sensors/PTT
  TT28 : Scope
  scope19 : Scope
  scope20 : Scope
  scope21 : Scope
  to_coldbox : PMIOPort  Port=1  Side=Left
  from_dewar : PMIOPort  Port=2  Side=Right
  wires:
  PS-Simulink Converter62/1 -> FT39/1
  PS-Simulink Converter66/1 -> scope19/1
  Bias13/1 -> Gain7/1
  PS-Simulink Converter57/1 -> Mux18/1
  PS-Simulink Converter56/1 -> FT42/1
  Gain7/1 -> Bias14/1
  Constant18/1 -> Simulink-PS Converter25/1
  PS-Simulink Converter61/1 -> Mux17/1
  Mux16/1 -> TT25/1
  PS-Simulink Converter63/1 -> Mux16/1
  Mux17/1 -> TT28/1
  Bias14/1 -> scope20/1, Simulink-PS Converter27/1
  PS-Simulink Converter58/1 -> Mux18/2
  Mux18/1 -> TT26/1
  Constant20/1 -> Simulink-PS Converter28/1
  PS-Simulink Converter64/1 -> Mux17/2
  Constant19/1 -> Simulink-PS Converter26/1
  PS-Simulink Converter60/1 -> FT38/1
  PS-Simulink Converter59/1 -> Mux16/2
  PS-Simulink Converter65/1 -> scope21/1, Bias13/1
  connections:
  PS-Simulink Converter60/LConn1 -- FT37/RConn1
  Simulink-PS Converter27/RConn1 -- FCV13/LConn1
  PS-Simulink Converter62/LConn1 -- FT41/RConn1
  M src21/RConn1 -- PhaseSep7/RConn3
  Simulink-PS Converter25/RConn1 -- PhaseSep7/RConn4
  PS-Simulink Converter56/LConn1 -- FT40/RConn1
  from_dewar/RConn1 -- Distributor13/LConn1
  FCV00 2 7/LConn2 -- Distributor13/RConn1
  FCV14/LConn2 -- PhaseSep7/LConn1 -- BP_out-E13/LConn1 -- FT41/LConn1
  BP_out-E13/RConn1 -- PS-Simulink Converter58/LConn1
  PS-Simulink Converter65/LConn1 -- PhaseSep7/RConn5
  PhaseSep7/LConn2 -- P/T src11/RConn1
  PhaseSep7/RConn2 -- M src20/RConn1
  Distributor13/RConn2 -- FCV13/LConn2
  TT27/RConn1 -- PS-Simulink Converter63/LConn1
  FT37/LConn1 -- TT27/LConn1 -- FCV00 2 7/RConn1 -- Mixer15/LConn1
  Simulink-PS Converter26/RConn1 -- FCV00 2 7/LConn1
  P/T src12/RConn1 -- PhaseSep7/LConn3
  M src19/RConn1 -- PhaseSep7/RConn1
  BP_out-E14/RConn1 -- PS-Simulink Converter64/LConn1
  TT27/RConn2 -- PS-Simulink Converter59/LConn1
  FCV14/LConn1 -- Simulink-PS Converter28/RConn1
  PS-Simulink Converter66/LConn1 -- PhaseSep7/LConn5
  BP_out-E13/RConn2 -- PS-Simulink Converter57/LConn1
  BP_out-E14/RConn2 -- PS-Simulink Converter61/LConn1
  FCV13/RConn1 -- Mixer15/LConn2 -- FT40/LConn1 -- BP_out-E14/LConn1
  PhaseSep7/LConn4 -- Mixer15/RConn1
  FCV14/RConn1 -- to_coldbox/RConn1

== system assemblage_19/Cryomodules/CMA8 ==
  BP_out-E15 : simCryogenics_lib/Sensors/PTT
  BP_out-E16 : simCryogenics_lib/Sensors/PTT
  Bias15 : Bias  Bias=-50
  Bias16 : Bias  Bias=100
  Constant21 : Constant  Value=W
  Constant22 : Constant  Value=0
  Constant23 : Constant  Value=63
  Distributor14 : simCryogenics_lib/Elements/Distributor2
  FCV00 2 8 : simCryogenics_lib/Elements/Valve  CVmax=0.2  ControlInputMin=0  ControlInputMax=100  Xt=0.86  Rv=100  lin_v=0  lim_v=0  K=2.4e-5 m^1.50000*kg^0.50000/s/bar^0.50000  Cmd_specify=off  Cmd_priority=High  Cmd=0  gamma_specify=off  gamma_priority=High  gamma=0  rho_specify=off  rho_priority=High  rho=0 kg/m^3  Xc_specify=off  Xc_priority=High  Xc=0  X_specify=off  X_priority=High  X=0  Y_specify=off  Y_priority=High  Y=0  CV_specify=off  CV_priority=High  CV=0
  FCV15 : simCryogenics_lib/Elements/Valve  CVmax=1.25  ControlInputMin=0  ControlInputMax=100  Xt=0.86  Rv=150  lin_v=0  lim_v=0  K=2.4e-5 m^1.50000*kg^0.50000/s/bar^0.50000  Cmd_specify=off  Cmd_priority=High  Cmd=0  gamma_specify=off  gamma_priority=High  gamma=0  rho_specify=off  rho_priority=High  rho=0 kg/m^3  Xc_specify=off  Xc_priority=High  Xc=0  X_specify=off  X_priority=High  X=0  Y_specify=off  Y_priority=High  Y=0  CV_specify=off  CV_priority=High  CV=0
  FCV16 : simCryogenics_lib/Elements/Valve  CVmax=1.5  ControlInputMin=0  ControlInputMax=100  Xt=0.86  Rv=100  lin_v=0  lim_v=0  K=2.4e-5 m^1.50000*kg^0.50000/s/bar^0.50000  Cmd_specify=off  Cmd_priority=High  Cmd=0  gamma_specify=off  gamma_priority=High  gamma=0  rho_specify=off  rho_priority=High  rho=0 kg/m^3  Xc_specify=off  Xc_priority=High  Xc=0  X_specify=off  X_priority=High  X=0  Y_specify=off  Y_priority=High  Y=0  CV_specify=off  CV_priority=High  CV=0
  FT43 : simCryogenics_lib/Sensors/FT
  FT44 : Scope
  FT45 : Scope
  FT46 : simCryogenics_lib/Sensors/FT
  FT47 : simCryogenics_lib/Sensors/FT
  FT48 : Scope
  Gain8 : Gain  Gain=-10
  M src22 : simCryogenics_lib/Sources_Sinks/M src  M=0 kg/s
  M src23 : simCryogenics_lib/Sources_Sinks/M src  M=0 kg/s
  M src24 : simCryogenics_lib/Sources_Sinks/M src  M=0 kg/s
  Mixer16 : simCryogenics_lib/Elements/Mixer2
  Mux19 : Mux  Inputs=2
  Mux20 : Mux  Inputs=2
  Mux21 : Mux  Inputs=2
  P/T src15 : simCryogenics_lib/Sources_Sinks/P//T src  P=1.2 bar  T=4.4 K
  P/T src16 : simCryogenics_lib/Sources_Sinks/P//T src  P=1.2 bar  T=4.4 K
  PS-Simulink Converter{67..77} (11 alike) : nesl_utility/PS-Simulink Converter  PhysicalDomain=network_engine_domain  SubClassName=ps_output  LeftPortType=input  RightPortType=output  PseudoPeriodic=off  Frequencies=[]  Unit=1  AffineConversion=off
  PhaseSep8 : simCryogenics_lib/Elements/PhaseSep  Ideal1=1  DeltaT1=0.05 K  N1=10  h1=400 W/K  Ideal2=1  DeltaT2=0.05 K  N2=10  h2=400 W/K  hmax=0.870 m  S=0.0402 m^2  P0=1.25 bar  h0=50  T0=4.5 K
  Simulink-PS Converter{29..32} (4 alike) : nesl_utility/Simulink-PS Converter  PhysicalDomain=network_engine_domain  SubClassName=ps_input  LeftPortType=input  RightPortType=output  PseudoPeriodic=off  Frequencies=[]  NoiseDistribution=none  NoiseParameters=[]  Unit=1  AffineConversion=off  InputFiltering=off  SimscapeFilterOrder=1  InputFilterTimeConstant=0.001  UdotUserProvided=1
  TT29 : Scope
  TT30 : Scope
  TT31 : simCryogenics_lib/Sensors/PTT
  TT32 : Scope
  scope22 : Scope
  scope23 : Scope
  scope24 : Scope
  to_coldbox : PMIOPort  Port=1  Side=Left
  from_dewar : PMIOPort  Port=2  Side=Right
  wires:
  Gain8/1 -> Bias16/1
  PS-Simulink Converter73/1 -> FT45/1
  Constant23/1 -> Simulink-PS Converter32/1
  PS-Simulink Converter72/1 -> Mux20/1
  PS-Simulink Converter77/1 -> scope22/1
  PS-Simulink Converter67/1 -> FT48/1
  Bias15/1 -> Gain8/1
  PS-Simulink Converter71/1 -> FT44/1
  Mux19/1 -> TT29/1
  Mux20/1 -> TT32/1
  Bias16/1 -> scope23/1, Simulink-PS Converter31/1
  Constant21/1 -> Simulink-PS Converter29/1
  Mux21/1 -> TT30/1
  PS-Simulink Converter70/1 -> Mux19/2
  PS-Simulink Converter68/1 -> Mux21/1
  Constant22/1 -> Simulink-PS Converter30/1
  PS-Simulink Converter76/1 -> scope24/1, Bias15/1
  PS-Simulink Converter74/1 -> Mux19/1
  PS-Simulink Converter75/1 -> Mux20/2
  PS-Simulink Converter69/1 -> Mux21/2
  connections:
  FCV00 2 8/LConn2 -- Distributor14/RConn1
  PS-Simulink Converter71/LConn1 -- FT43/RConn1
  TT31/RConn1 -- PS-Simulink Converter74/LConn1
  M src22/RConn1 -- PhaseSep8/RConn1
  BP_out-E15/RConn2 -- PS-Simulink Converter68/LConn1
  Simulink-PS Converter29/RConn1 -- PhaseSep8/RConn4
  TT31/RConn2 -- PS-Simulink Converter70/LConn1
  M src24/RConn1 -- PhaseSep8/RConn3
  FCV16/LConn1 -- Simulink-PS Converter32/RConn1
  PhaseSep8/RConn2 -- M src23/RConn1
  PhaseSep8/LConn4 -- Mixer16/RConn1
  FT43/LConn1 -- TT31/LConn1 -- FCV00 2 8/RConn1 -- Mixer16/LConn1
  P/T src16/RConn1 -- PhaseSep8/LConn3
  PS-Simulink Converter67/LConn1 -- FT46/RConn1
  FCV16/LConn2 -- PhaseSep8/LConn1 -- BP_out-E15/LConn1 -- FT47/LConn1
  from_dewar/RConn1 -- Distributor14/LConn1
  FCV15/RConn1 -- Mixer16/LConn2 -- FT46/LConn1 -- BP_out-E16/LConn1
  BP_out-E16/RConn2 -- PS-Simulink Converter72/LConn1
  FCV16/RConn1 -- to_coldbox/RConn1
  PhaseSep8/LConn2 -- P/T src15/RConn1
  PS-Simulink Converter73/LConn1 -- FT47/RConn1
  Simulink-PS Converter30/RConn1 -- FCV00 2 8/LConn1
  PS-Simulink Converter77/LConn1 -- PhaseSep8/LConn5
  PS-Simulink Converter76/LConn1 -- PhaseSep8/RConn5
  BP_out-E15/RConn1 -- PS-Simulink Converter69/LConn1
  Simulink-PS Converter31/RConn1 -- FCV15/LConn1
  Distributor14/RConn2 -- FCV15/LConn2
  BP_out-E16/RConn1 -- PS-Simulink Converter75/LConn1

== system assemblage_19/Cryomodules/CMA9 ==
  BP_out-E17 : simCryogenics_lib/Sensors/PTT
  BP_out-E18 : simCryogenics_lib/Sensors/PTT
  Bias17 : Bias  Bias=-50
  Bias18 : Bias  Bias=100
  Constant24 : Constant  Value=W
  Constant25 : Constant  Value=0
  Constant26 : Constant  Value=63
  Distributor15 : simCryogenics_lib/Elements/Distributor2
  FCV00 2 9 : simCryogenics_lib/Elements/Valve  CVmax=0.2  ControlInputMin=0  ControlInputMax=100  Xt=0.86  Rv=100  lin_v=0  lim_v=0  K=2.4e-5 m^1.50000*kg^0.50000/s/bar^0.50000  Cmd_specify=off  Cmd_priority=High  Cmd=0  gamma_specify=off  gamma_priority=High  gamma=0  rho_specify=off  rho_priority=High  rho=0 kg/m^3  Xc_specify=off  Xc_priority=High  Xc=0  X_specify=off  X_priority=High  X=0  Y_specify=off  Y_priority=High  Y=0  CV_specify=off  CV_priority=High  CV=0
  FCV17 : simCryogenics_lib/Elements/Valve  CVmax=1.25  ControlInputMin=0  ControlInputMax=100  Xt=0.86  Rv=150  lin_v=0  lim_v=0  K=2.4e-5 m^1.50000*kg^0.50000/s/bar^0.50000  Cmd_specify=off  Cmd_priority=High  Cmd=0  gamma_specify=off  gamma_priority=High  gamma=0  rho_specify=off  rho_priority=High  rho=0 kg/m^3  Xc_specify=off  Xc_priority=High  Xc=0  X_specify=off  X_priority=High  X=0  Y_specify=off  Y_priority=High  Y=0  CV_specify=off  CV_priority=High  CV=0
  FCV18 : simCryogenics_lib/Elements/Valve  CVmax=1.5  ControlInputMin=0  ControlInputMax=100  Xt=0.86  Rv=100  lin_v=0  lim_v=0  K=2.4e-5 m^1.50000*kg^0.50000/s/bar^0.50000  Cmd_specify=off  Cmd_priority=High  Cmd=0  gamma_specify=off  gamma_priority=High  gamma=0  rho_specify=off  rho_priority=High  rho=0 kg/m^3  Xc_specify=off  Xc_priority=High  Xc=0  X_specify=off  X_priority=High  X=0  Y_specify=off  Y_priority=High  Y=0  CV_specify=off  CV_priority=High  CV=0
  FT49 : simCryogenics_lib/Sensors/FT
  FT50 : Scope
  FT51 : Scope
  FT52 : simCryogenics_lib/Sensors/FT
  FT53 : simCryogenics_lib/Sensors/FT
  FT54 : Scope
  Gain9 : Gain  Gain=-10
  M src25 : simCryogenics_lib/Sources_Sinks/M src  M=0 kg/s
  M src26 : simCryogenics_lib/Sources_Sinks/M src  M=0 kg/s
  M src27 : simCryogenics_lib/Sources_Sinks/M src  M=0 kg/s
  Mixer17 : simCryogenics_lib/Elements/Mixer2
  Mux22 : Mux  Inputs=2
  Mux23 : Mux  Inputs=2
  Mux24 : Mux  Inputs=2
  P/T src17 : simCryogenics_lib/Sources_Sinks/P//T src  P=1.2 bar  T=4.4 K
  P/T src18 : simCryogenics_lib/Sources_Sinks/P//T src  P=1.2 bar  T=4.4 K
  PS-Simulink Converter{78..88} (11 alike) : nesl_utility/PS-Simulink Converter  PhysicalDomain=network_engine_domain  SubClassName=ps_output  LeftPortType=input  RightPortType=output  PseudoPeriodic=off  Frequencies=[]  Unit=1  AffineConversion=off
  PhaseSep9 : simCryogenics_lib/Elements/PhaseSep  Ideal1=1  DeltaT1=0.05 K  N1=10  h1=400 W/K  Ideal2=1  DeltaT2=0.05 K  N2=10  h2=400 W/K  hmax=0.870 m  S=0.0402 m^2  P0=1.25 bar  h0=50  T0=4.5 K
  Simulink-PS Converter{33..36} (4 alike) : nesl_utility/Simulink-PS Converter  PhysicalDomain=network_engine_domain  SubClassName=ps_input  LeftPortType=input  RightPortType=output  PseudoPeriodic=off  Frequencies=[]  NoiseDistribution=none  NoiseParameters=[]  Unit=1  AffineConversion=off  InputFiltering=off  SimscapeFilterOrder=1  InputFilterTimeConstant=0.001  UdotUserProvided=1
  TT33 : Scope
  TT34 : Scope
  TT35 : simCryogenics_lib/Sensors/PTT
  TT36 : Scope
  scope25 : Scope
  scope26 : Scope
  scope27 : Scope
  to_coldbox : PMIOPort  Port=1  Side=Left
  from_dewar : PMIOPort  Port=2  Side=Right
  wires:
  Gain9/1 -> Bias18/1
  PS-Simulink Converter87/1 -> scope27/1, Bias17/1
  PS-Simulink Converter84/1 -> FT51/1
  Constant25/1 -> Simulink-PS Converter34/1
  PS-Simulink Converter83/1 -> Mux23/1
  Constant26/1 -> Simulink-PS Converter36/1
  PS-Simulink Converter79/1 -> Mux24/1
  Bias18/1 -> scope26/1, Simulink-PS Converter35/1
  PS-Simulink Converter88/1 -> scope25/1
  Constant24/1 -> Simulink-PS Converter33/1
  PS-Simulink Converter86/1 -> Mux23/2
  PS-Simulink Converter82/1 -> FT50/1
  Mux22/1 -> TT33/1
  PS-Simulink Converter80/1 -> Mux24/2
  Mux24/1 -> TT34/1
  Mux23/1 -> TT36/1
  PS-Simulink Converter78/1 -> FT54/1
  PS-Simulink Converter85/1 -> Mux22/1
  PS-Simulink Converter81/1 -> Mux22/2
  Bias17/1 -> Gain9/1
  connections:
  M src25/RConn1 -- PhaseSep9/RConn1
  FCV00 2 9/LConn2 -- Distributor15/RConn1
  PhaseSep9/LConn2 -- P/T src17/RConn1
  PhaseSep9/RConn2 -- M src26/RConn1
  FT49/LConn1 -- TT35/LConn1 -- FCV00 2 9/RConn1 -- Mixer17/LConn1
  from_dewar/RConn1 -- Distributor15/LConn1
  BP_out-E18/RConn1 -- PS-Simulink Converter86/LConn1
  M src27/RConn1 -- PhaseSep9/RConn3
  P/T src18/RConn1 -- PhaseSep9/LConn3
  Simulink-PS Converter35/RConn1 -- FCV17/LConn1
  PhaseSep9/LConn4 -- Mixer17/RConn1
  TT35/RConn2 -- PS-Simulink Converter81/LConn1
  BP_out-E18/RConn2 -- PS-Simulink Converter83/LConn1
  PS-Simulink Converter78/LConn1 -- FT52/RConn1
  Distributor15/RConn2 -- FCV17/LConn2
  FCV18/LConn2 -- PhaseSep9/LConn1 -- BP_out-E17/LConn1 -- FT53/LConn1
  Simulink-PS Converter33/RConn1 -- PhaseSep9/RConn4
  PS-Simulink Converter88/LConn1 -- PhaseSep9/LConn5
  BP_out-E17/RConn1 -- PS-Simulink Converter80/LConn1
  BP_out-E17/RConn2 -- PS-Simulink Converter79/LConn1
  PS-Simulink Converter87/LConn1 -- PhaseSep9/RConn5
  PS-Simulink Converter84/LConn1 -- FT53/RConn1
  FCV18/LConn1 -- Simulink-PS Converter36/RConn1
  FCV18/RConn1 -- to_coldbox/RConn1
  FCV17/RConn1 -- Mixer17/LConn2 -- FT52/LConn1 -- BP_out-E18/LConn1
  Simulink-PS Converter34/RConn1 -- FCV00 2 9/LConn1
  PS-Simulink Converter82/LConn1 -- FT49/RConn1
  TT35/RConn1 -- PS-Simulink Converter85/LConn1
